simulink library "ss_vec_2_angles"  (R2016b)
settings: Solver=VariableStepAuto  StartTime=0.0  StopTime=10.0  RelTol=1e-3
settings Model: Creator=taylorreynolds  LastModifiedBy=Taylor

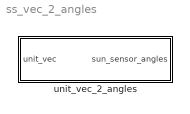
== system ss_vec_2_angles ==
  unit_vec_2_angles : Subsystem

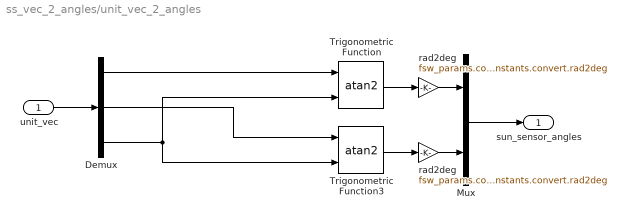
== system ss_vec_2_angles/unit_vec_2_angles ==
  unit_vec : Inport
  Demux : Demux  Outputs=3
  Mux : Mux  Inputs=2
  Trigonometric Function : Trigonometry  Operator=atan2
  Trigonometric Function3 : Trigonometry  Operator=atan2
  rad2deg : Gain  Gain=fsw_params.constants.convert.rad2deg
  "rad2deg " : Gain  Gain=fsw_params.constants.convert.rad2deg
  sun_sensor_angles : Outport
  wires:
  Trigonometric Function3/1 -> "rad2deg "/1
  unit_vec/1 -> Demux/1
  Demux/2 -> Trigonometric Function3/1
  Trigonometric Function/1 -> rad2deg/1
  Mux/1 -> sun_sensor_angles/1
  rad2deg/1 -> Mux/1
  "rad2deg "/1 -> Mux/2
  Demux/1 -> Trigonometric Function/1
  Demux/3 -> Trigonometric Function/2, Trigonometric Function3/2
